simulink model "MOSSE_HDL_final"  (Simulink 8.3)
settings: Solver=FixedStepDiscrete  SolverMode=SingleTasking  StartTime=0.0  StopTime=30*640*360  RelTol=1e-3
InitFcn:
  | %% DSPBuilder Start
  | alt_dspbuilder_update_model(bdroot)
  | %% DSPBuilder End
  | param
StopFcn:
  | % r = rcount.Data(:,:);
  | % w = wcount.Data(:,:);
  | % d = dout.Data(:,:);
  | % ir = read.Data(:,:);
  | % iw = write.Data(:,:);
  | % z = double([ir iw d r w]');
  | %logic_analyzer
values from neighbouring files (symbols this model uses):
  Gau = [4035 -3983 3832 -3589 3269 -2890 2472 -2039 1612 -1211 854 -553 ... (4096 elements, 1x4096)]    [Gauss_coeff.mat]    (also in param.m = reshape(conj(Gau'), 1, 4096))
undefined symbols (not defined in the file or in its folder): gray, psr, source_1, source_2, State_Machine, State_Transition_Table1, window_hann
libraries: allblocks_alteradspbuilder2 x166, hdlsllib x24, hdldemolib x3, simulink x2, dspsigattribs x2, dspmtrx3 x2, visionsinks x1, visiontextngfix x1, dspvision x1
(part 1 of 4)
settings Model: FPTRunName=FPA_Reference  Creator=minimal  LastModifiedBy=minimales
settings DataIOCC: SignalLoggingSaveFormat=Dataset
settings HardwareCC: ProdHWDeviceType=ASIC/FPGA->ASIC/FPGA  TargetIntDivRoundTo=Zero  TargetEndianess=LittleEndian  TargetHWDeviceType=MATLAB Host  ProdEqTarget=off
settings GRTTargetCC: CombineOutputUpdateFcns=on  GRTInterface=off

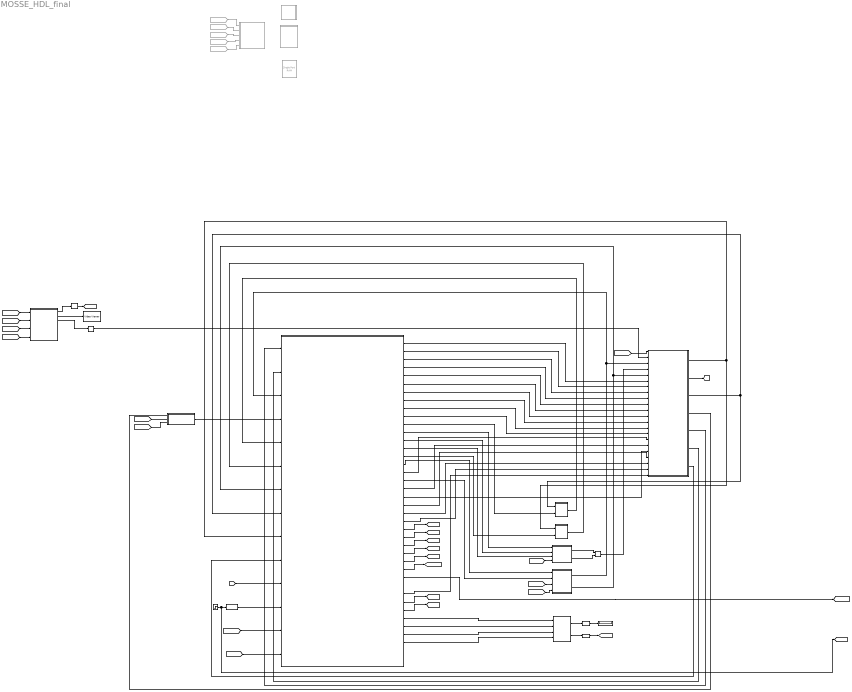
== system MOSSE_HDL_final ==
  DSP_Buider_Alfa_blending_H1 : Subsystem
  DSP_Builder_Alfa_blending_H2 : Subsystem
  DSP_Builder_Compute_PSR : Subsystem  Commented=on
  DSP_Builder_Compute_Shift : Subsystem  Commented=on
  DSP_Builder_Divider Complex : Subsystem
  DSP_Builder_Mult_complex : Subsystem
  DSP_Builder_PSR : Subsystem
  DSP_Builder_Smoothing_Window : Subsystem
  Data Type Conversion1 : DataTypeConversion  OutDataTypeStr=boolean
  Data Type Conversion19 : DataTypeConversion  OutDataTypeStr=int16
  Data Type Conversion5 : DataTypeConversion  OutDataTypeStr=boolean  SampleTime=1
  Delay : Delay  DelayLength=1  InitialCondition=0  SampleTime=1
  Delay1 : Delay  DelayLength=1  InitialCondition=0  SampleTime=1
  Display1 : Display
  From38 : From  Commented=on  GotoTag=source_enb
  From39 : From  Commented=on  GotoTag=source1_enb
  From40 : From  Commented=on  GotoTag=source_control
  From41 : From  Commented=on  GotoTag=source_count_enb
  From42 : From  Commented=on  GotoTag=source_count_rst
  HDL_CODER_Subsystem : Subsystem
  IFFT_res : hdlsllib/HDL Operations/Single Port RAM  Commented=on  ram_size=12  dout_type=New data
  MEM_subsys : Subsystem
  Real-Imag to Complex : RealImagToComplex
  Source : Subsystem  Commented=on
  Step1 : Step  SampleTime=1
  Video Viewer1 : visionsinks/Video Viewer  inputType=Obsolete7b  imagePorts=One multidimensional signal  useColorMap=off  colormapValue=gray(256)  specRange=off  minInputVal=0  maxInputVal=255  FigPos=[1 992 1280 892]  AxisZoom=on  trueSizedOnce=off  OpenAtMdlStart=on  DefaultConfigurationName=vipscopes.VideoViewerScopeCfg
  Video_TestBench : Subsystem
  wires:
  DSP_Builder_Divider Complex/2(Im_r) -> Real-Imag to Complex/2
  DSP_Builder_Divider Complex/1(Re_r) -> Real-Imag to Complex/1
  [rst_win] -> DSP_Builder_Smoothing_Window/2(rst)
  [enb_win] -> DSP_Builder_Smoothing_Window/3(enb)
  [div_complex_aclr] -> DSP_Builder_Divider Complex/4(aclr_i)
  [rst_gauss] -> DSP_Builder_Mult_complex/3(rst)
  [enb_gauss] -> DSP_Builder_Mult_complex/4(enb)
  DSP_Builder_PSR/2(psr_check) -> Data Type Conversion1/1
  Data Type Conversion19/1 -> Display1/1
  Step1/1 -> [enable_tracking], Data Type Conversion5/1
  DSP_Builder_Mult_complex/1(H2) -> MEM_subsys/3(wr_din_F_RAM), HDL_CODER_Subsystem/3("H2 ")
  DSP_Builder_Mult_complex/2(H1) -> MEM_subsys/5(wr_din_G_RAM), HDL_CODER_Subsystem/7(H1)
  DSP_Builder_Smoothing_Window/1(opixel) -> HDL_CODER_Subsystem/4(iPixel_image)
  DSP_Buider_Alfa_blending_H1/1(H) -> HDL_CODER_Subsystem/5(H1_alfa)
  DSP_Builder_Alfa_blending_H2/1(H) -> HDL_CODER_Subsystem/6(H2_alfa)
  [Corr] -> HDL_CODER_Subsystem/11(iCorr_data)
  Data Type Conversion5/1 -> HDL_CODER_Subsystem/12(enable_Tracking)
  [psr_check] -> HDL_CODER_Subsystem/13(psr_check)
  HDL_CODER_Subsystem/11(oData1) -> DSP_Buider_Alfa_blending_H1/2(H_n)
  HDL_CODER_Subsystem/12(Real_H1) -> DSP_Builder_Divider Complex/1(Re_a)
  HDL_CODER_Subsystem/13(Real_H2) -> DSP_Builder_Divider Complex/2(Re_b)
  HDL_CODER_Subsystem/14(Imag_H1) -> DSP_Builder_Divider Complex/3(Im_a)
  HDL_CODER_Subsystem/15(oData2) -> DSP_Builder_Alfa_blending_H2/2(H_n)
  HDL_CODER_Subsystem/16(oF*) -> DSP_Builder_Mult_complex/1(F*)
  HDL_CODER_Subsystem/18(oF) -> DSP_Builder_Mult_complex/2(F)
  HDL_CODER_Subsystem/24(addr_memory_128x128) -> [mem_addr]
  HDL_CODER_Subsystem/25(rst_win) -> [rst_win]
  HDL_CODER_Subsystem/26(enb_win) -> [enb_win]
  HDL_CODER_Subsystem/27(rst_gauss) -> [rst_gauss]
  HDL_CODER_Subsystem/28(enb_gauss) -> [enb_gauss]
  HDL_CODER_Subsystem/29(div_complex) -> [div_complex_aclr]
  HDL_CODER_Subsystem/30(comp_shift_finish) -> [comp_shift_finish]
  [enable_tracking] -> Video_TestBench/1(en)
  [comp_shift_finish] -> Video_TestBench/4(comp_shift_finish)
  Video_TestBench/2(video_viewer) -> Video Viewer1/1
  From40/1 -> Source/1(source_control)
  From38/1 -> Source/2(source_enb)
  From42/1 -> Source/3(source_count_rst)
  From41/1 -> Source/4(source_count_enb)
  From39/1 -> Source/5(source1_enb)
  [enable_write] -> HDL_CODER_Subsystem/14(enable_write)
  [dx] -> Video_TestBench/2(dx)
  [dy] -> Video_TestBench/3(dy)
  Video_TestBench/1(enable_write) -> Delay/1
  Video_TestBench/3(serialized_data) -> Delay1/1
  DSP_Builder_PSR/1(psr) -> Data Type Conversion19/1
  MEM_subsys/3(rd_dout_H1_RAM) -> DSP_Buider_Alfa_blending_H1/1(H_p), HDL_CODER_Subsystem/8(H1_p)
  MEM_subsys/1(rd_dout_H2_RAM) -> DSP_Builder_Alfa_blending_H2/1(H_p), HDL_CODER_Subsystem/9(H2_p)
  [mem_addr] -> MEM_subsys/1(rd_addr_Ext_im_RAM)
  Delay1/1 -> MEM_subsys/2(wr_din_Ext_im_RAM)
  Real-Imag to Complex/1 -> MEM_subsys/4(wr_din_H_RAM)
  HDL_CODER_Subsystem/1(oH2) -> MEM_subsys/6(wr_din_H2_RAM)
  HDL_CODER_Subsystem/2(wr_addr_H1_H2) -> MEM_subsys/7(wr_addr_H1_H2_RAM)
  HDL_CODER_Subsystem/3(we_H1_H2) -> MEM_subsys/8(wr_en_H1_H2_RAM)
  HDL_CODER_Subsystem/4(wr_addr_G_F) -> MEM_subsys/9(wr_addr_G_F_RAM)
  HDL_CODER_Subsystem/5(we_G_F) -> MEM_subsys/10(wr_en_G_F_RAM)
  HDL_CODER_Subsystem/6(addr_in_im) -> MEM_subsys/11(wr_addr_Ext_im_RAM)
  HDL_CODER_Subsystem/7(rd_addr_H1_H2) -> MEM_subsys/12(rd_addr_H1_H2_RAM)
  HDL_CODER_Subsystem/8(rd_addr_G_F) -> MEM_subsys/13(rd_addr_G_F_RAM)
  HDL_CODER_Subsystem/9(we_m) -> MEM_subsys/14(wr_en_Ext_im_RAM)
  HDL_CODER_Subsystem/10(oH1) -> MEM_subsys/15(wr_din_H1_RAM)
  HDL_CODER_Subsystem/17(wr_addr_H) -> MEM_subsys/16(wr_addr_H_RAM)
  HDL_CODER_Subsystem/19(we_H) -> MEM_subsys/17(wr_en_H_RAM)
  HDL_CODER_Subsystem/20(rd_addr_H) -> MEM_subsys/18(rd_addr_H_RAM)
  HDL_CODER_Subsystem/21(RAM_data) -> MEM_subsys/19(wr_din_IFFT_res_RAM)
  HDL_CODER_Subsystem/22(wr_addr_RAM_IFFT) -> MEM_subsys/20(wr_addr_IFFT_res_RAM)
  HDL_CODER_Subsystem/23(we_RAM_IFFT) -> MEM_subsys/21(wr_en_IFFT_res_RAM)
  HDL_CODER_Subsystem/32(rd_addr_RAM_IFFT) -> MEM_subsys/22(rd_addr_IFFT_res_RAM)
  MEM_subsys/2(rd_dout_H_RAM) -> [Corr]
  MEM_subsys/4(rd_dout_Ext_im_RAM) -> DSP_Builder_Smoothing_Window/1(ipixel)
  MEM_subsys/5(rd_dout_G_RAM) -> HDL_CODER_Subsystem/1(G)
  MEM_subsys/6(rd_dout_F_RAM) -> HDL_CODER_Subsystem/2(F)
  MEM_subsys/7(rd_dout_IFFT_res_RAM) -> HDL_CODER_Subsystem/10(In12)
  HDL_CODER_Subsystem/33(Dx) -> [dx]
  HDL_CODER_Subsystem/34(Dy) -> [dy]
  HDL_CODER_Subsystem/35(max_val) -> DSP_Builder_PSR/1(max)
  HDL_CODER_Subsystem/36(mean_val) -> DSP_Builder_PSR/2(mean)
  HDL_CODER_Subsystem/37(tmp_val) -> DSP_Builder_PSR/3(tmp)
  Delay/1 -> [enable_write]
  HDL_CODER_Subsystem/38(psr_reset) -> DSP_Builder_PSR/4(psr_reset)
  Data Type Conversion1/1 -> [psr_check]

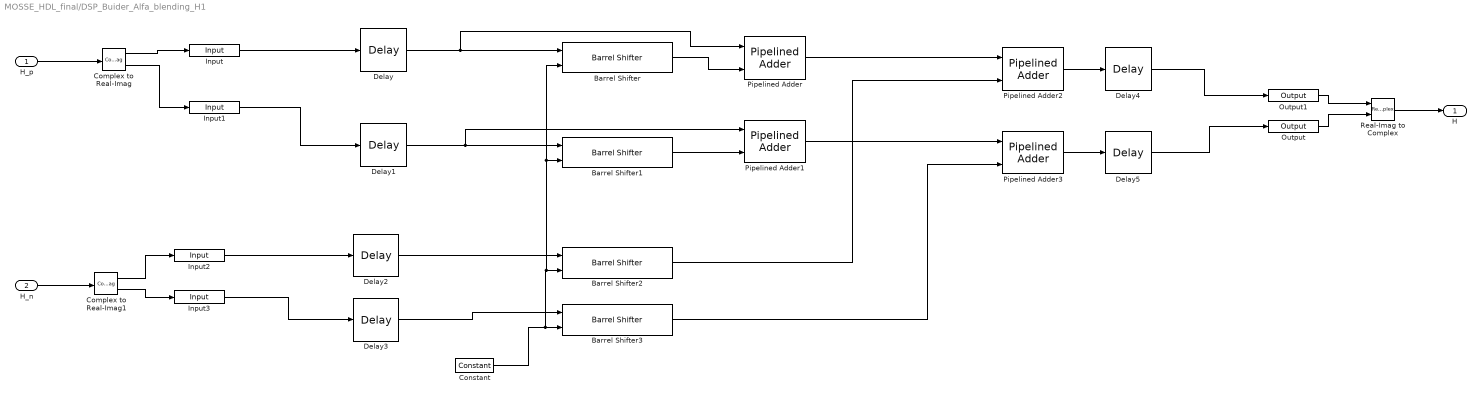
== system MOSSE_HDL_final/DSP_Buider_Alfa_blending_H1 ==
  H_p : Inport
  H_n : Inport  Port=2
  Barrel Shifter : allblocks_alteradspbuilder2/Barrel Shifter  BusType=Signed Integer  bwl=32  bwr=8  pipeline=off  infer_distance=off  distance_length=3  ShiftDirection=Shift right  use_ena=off  use_aclr=off  UseDedicatedCircuitry=off  pipeline_display=0  allowFloatingPointOverride=on  logOutputs=off  logFile=C:\MOSSE%5FHDL%5Ffinal_DSP%5FBuider%5FAlfa%5Fblending%5FH1_Barrel+Shifter.fixedpointlog
  Barrel Shifter1 : allblocks_alteradspbuilder2/Barrel Shifter  BusType=Signed Integer  bwl=32  bwr=8  pipeline=off  infer_distance=off  distance_length=3  ShiftDirection=Shift right  use_ena=off  use_aclr=off  UseDedicatedCircuitry=off  pipeline_display=0  allowFloatingPointOverride=on  logOutputs=off  logFile=E:\Work\ComputerVision\ObjectTrack\MOSSE\autotrackigproject\Model\MOSSE_algorithm\MOSSE_simulink\tb_MOSSE_HDL_final\MOSSE%5FHDL%5Ffinal_DSP%5FBuider%5FAlfa%5Fblending%5FH1_Barrel+Shifter1.fixedpointlog
  Barrel Shifter2 : allblocks_alteradspbuilder2/Barrel Shifter  BusType=Signed Integer  bwl=32  bwr=8  pipeline=off  infer_distance=off  distance_length=3  ShiftDirection=Shift right  use_ena=off  use_aclr=off  UseDedicatedCircuitry=off  pipeline_display=0  allowFloatingPointOverride=on  logOutputs=off  logFile=E:\Work\ComputerVision\ObjectTrack\MOSSE\autotrackigproject\Model\MOSSE_algorithm\MOSSE_simulink\tb_MOSSE_HDL_final\MOSSE%5FHDL%5Ffinal_DSP%5FBuider%5FAlfa%5Fblending%5FH1_Barrel+Shifter2.fixedpointlog
  Barrel Shifter3 : allblocks_alteradspbuilder2/Barrel Shifter  BusType=Signed Integer  bwl=32  bwr=8  pipeline=off  infer_distance=off  distance_length=3  ShiftDirection=Shift right  use_ena=off  use_aclr=off  UseDedicatedCircuitry=off  pipeline_display=0  allowFloatingPointOverride=on  logOutputs=off  logFile=E:\Work\ComputerVision\ObjectTrack\MOSSE\autotrackigproject\Model\MOSSE_algorithm\MOSSE_simulink\tb_MOSSE_HDL_final\MOSSE%5FHDL%5Ffinal_DSP%5FBuider%5FAlfa%5Fblending%5FH1_Barrel+Shifter3.fixedpointlog
  Complex to Real-Imag : ComplexToRealImag
  Complex to Real-Imag1 : ComplexToRealImag
  Constant : allblocks_alteradspbuilder2/Constant  mask_cst=K_shift  BusType=Unsigned Integer  bwl=3  bwr=0  roundMode=Truncate  satMode=Wrap  SpecifyClock=off  allowFloatingPointOverride=on  logOutputs=off  logFile=E:\Work\ComputerVision\ObjectTrack\MOSSE\autotrackigproject\Model\MOSSE_algorithm\MOSSE_simulink\tb_MOSSE_HDL_final\MOSSE%5FHDL%5Ffinal_DSP%5FBuider%5FAlfa%5Fblending%5FH1_Constant.fixedpointlog
  Delay : allblocks_alteradspbuilder2/Delay  pipeline=1  pipeline_display=1  ClockPhase=1  use_ena=off  use_sclr=off  allowFloatingPointOverride=on  logOutputs=off  logFile=E:\Work\ComputerVision\ObjectTrack\MOSSE\autotrackigproject\Model\MOSSE_algorithm\MOSSE_simulink\tb_MOSSE_HDL_final\MOSSE%5FHDL%5Ffinal_DSP%5FBuider%5FAlfa%5Fblending%5FH1_Delay.fixedpointlog  use_init=off  reset_value=1
  Delay1 : allblocks_alteradspbuilder2/Delay  pipeline=1  pipeline_display=1  ClockPhase=1  use_ena=off  use_sclr=off  allowFloatingPointOverride=on  logOutputs=off  logFile=E:\Work\ComputerVision\ObjectTrack\MOSSE\autotrackigproject\Model\MOSSE_algorithm\MOSSE_simulink\tb_MOSSE_HDL_final\MOSSE%5FHDL%5Ffinal_DSP%5FBuider%5FAlfa%5Fblending%5FH1_Delay1.fixedpointlog  use_init=off  reset_value=1
  Delay2 : allblocks_alteradspbuilder2/Delay  pipeline=1  pipeline_display=1  ClockPhase=1  use_ena=off  use_sclr=off  allowFloatingPointOverride=on  logOutputs=off  logFile=E:\Work\ComputerVision\ObjectTrack\MOSSE\autotrackigproject\Model\MOSSE_algorithm\MOSSE_simulink\tb_MOSSE_HDL_final\MOSSE%5FHDL%5Ffinal_DSP%5FBuider%5FAlfa%5Fblending%5FH1_Delay2.fixedpointlog  use_init=off  reset_value=1
  Delay3 : allblocks_alteradspbuilder2/Delay  pipeline=1  pipeline_display=1  ClockPhase=1  use_ena=off  use_sclr=off  allowFloatingPointOverride=on  logOutputs=off  logFile=E:\Work\ComputerVision\ObjectTrack\MOSSE\autotrackigproject\Model\MOSSE_algorithm\MOSSE_simulink\tb_MOSSE_HDL_final\MOSSE%5FHDL%5Ffinal_DSP%5FBuider%5FAlfa%5Fblending%5FH1_Delay3.fixedpointlog  use_init=off  reset_value=1
  Delay4 : allblocks_alteradspbuilder2/Delay  pipeline=1  pipeline_display=1  ClockPhase=1  use_ena=off  use_sclr=off  allowFloatingPointOverride=on  logOutputs=off  logFile=E:\Work\ComputerVision\ObjectTrack\MOSSE\autotrackigproject\Model\MOSSE_algorithm\MOSSE_simulink\tb_MOSSE_HDL_final\MOSSE%5FHDL%5Ffinal_DSP%5FBuider%5FAlfa%5Fblending%5FH1_Delay4.fixedpointlog  use_init=off  reset_value=1
  Delay5 : allblocks_alteradspbuilder2/Delay  pipeline=1  pipeline_display=1  ClockPhase=1  use_ena=off  use_sclr=off  allowFloatingPointOverride=on  logOutputs=off  logFile=E:\Work\ComputerVision\ObjectTrack\MOSSE\autotrackigproject\Model\MOSSE_algorithm\MOSSE_simulink\tb_MOSSE_HDL_final\MOSSE%5FHDL%5Ffinal_DSP%5FBuider%5FAlfa%5Fblending%5FH1_Delay5.fixedpointlog  use_init=off  reset_value=1
  Input : allblocks_alteradspbuilder2/Input  iofile=E:\Work\ComputerVision\ObjectTrack\MOSSE\autotrackigproject\Model\MOSSE_algorithm\MOSSE_simulink\tb_MOSSE_HDL_final\MOSSE%5FHDL%5Ffinal_DSP%5FBuider%5FAlfa%5Fblending%5FH1_Input.salt  BusType=Signed Integer  bwl=32  bwr=0  SpecifyClock=off  PORTTYPE=Input  externalType=Inferred  allowFloatingPointOverride=on  logOutputs=off
  Input1 : allblocks_alteradspbuilder2/Input  iofile=E:\Work\ComputerVision\ObjectTrack\MOSSE\autotrackigproject\Model\MOSSE_algorithm\MOSSE_simulink\tb_MOSSE_HDL_final\MOSSE%5FHDL%5Ffinal_DSP%5FBuider%5FAlfa%5Fblending%5FH1_Input1.salt  BusType=Signed Integer  bwl=32  bwr=0  SpecifyClock=off  PORTTYPE=Input  externalType=Inferred  allowFloatingPointOverride=on  logOutputs=off
  Input2 : allblocks_alteradspbuilder2/Input  iofile=E:\Work\ComputerVision\ObjectTrack\MOSSE\autotrackigproject\Model\MOSSE_algorithm\MOSSE_simulink\tb_MOSSE_HDL_final\MOSSE%5FHDL%5Ffinal_DSP%5FBuider%5FAlfa%5Fblending%5FH1_Input2.salt  BusType=Signed Integer  bwl=32  bwr=0  SpecifyClock=off  PORTTYPE=Input  externalType=Inferred  allowFloatingPointOverride=on  logOutputs=off
  Input3 : allblocks_alteradspbuilder2/Input  iofile=E:\Work\ComputerVision\ObjectTrack\MOSSE\autotrackigproject\Model\MOSSE_algorithm\MOSSE_simulink\tb_MOSSE_HDL_final\MOSSE%5FHDL%5Ffinal_DSP%5FBuider%5FAlfa%5Fblending%5FH1_Input3.salt  BusType=Signed Integer  bwl=32  bwr=0  SpecifyClock=off  PORTTYPE=Input  externalType=Inferred  allowFloatingPointOverride=on  logOutputs=off
  Output : allblocks_alteradspbuilder2/Output  iofile=E:\Work\ComputerVision\ObjectTrack\MOSSE\autotrackigproject\Model\MOSSE_algorithm\MOSSE_simulink\tb_MOSSE_HDL_final\MOSSE%5FHDL%5Ffinal_DSP%5FBuider%5FAlfa%5Fblending%5FH1_Output.capture  BusType=Signed Integer  bwl=32  bwr=0  externalType=Simulink Fixed Point Type  PORTTYPE=Output  allowFloatingPointOverride=on  logOutputs=off
  Output1 : allblocks_alteradspbuilder2/Output  iofile=E:\Work\ComputerVision\ObjectTrack\MOSSE\autotrackigproject\Model\MOSSE_algorithm\MOSSE_simulink\tb_MOSSE_HDL_final\MOSSE%5FHDL%5Ffinal_DSP%5FBuider%5FAlfa%5Fblending%5FH1_Output1.capture  BusType=Signed Integer  bwl=32  bwr=0  externalType=Simulink Fixed Point Type  PORTTYPE=Output  allowFloatingPointOverride=on  logOutputs=off
  Pipelined Adder : allblocks_alteradspbuilder2/Pipelined Adder  BusType=Signed Integer  bwl=32  bwr=0  pipeline=0  pipeline_display=0  AddSubDirection=SUB  use_cin=off  use_ovl=off  use_addsub=off  use_ena=off  use_aclr=off  or_aclr_inputs=on
  Pipelined Adder1 : allblocks_alteradspbuilder2/Pipelined Adder  BusType=Signed Integer  bwl=32  bwr=0  pipeline=0  pipeline_display=0  AddSubDirection=SUB  use_cin=off  use_ovl=off  use_addsub=off  use_ena=off  use_aclr=off  or_aclr_inputs=on
  Pipelined Adder2 : allblocks_alteradspbuilder2/Pipelined Adder  BusType=Signed Integer  bwl=32  bwr=0  pipeline=0  pipeline_display=0  AddSubDirection=ADD  use_cin=off  use_ovl=off  use_addsub=off  use_ena=off  use_aclr=off  or_aclr_inputs=on
  Pipelined Adder3 : allblocks_alteradspbuilder2/Pipelined Adder  BusType=Signed Integer  bwl=32  bwr=0  pipeline=0  pipeline_display=0  AddSubDirection=ADD  use_cin=off  use_ovl=off  use_addsub=off  use_ena=off  use_aclr=off  or_aclr_inputs=on
  Real-Imag to Complex : RealImagToComplex
  H : Outport
  wires:
  Pipelined Adder/1 -> Pipelined Adder2/1
  Barrel Shifter/1 -> Pipelined Adder/2
  Barrel Shifter2/1 -> Pipelined Adder2/2
  Barrel Shifter3/1 -> Pipelined Adder3/2
  Pipelined Adder1/1 -> Pipelined Adder3/1
  Barrel Shifter1/1 -> Pipelined Adder1/2
  H_p/1 -> Complex to Real-Imag/1
  H_n/1 -> Complex to Real-Imag1/1
  Real-Imag to Complex/1 -> H/1
  Constant/1 -> Barrel Shifter/2, Barrel Shifter1/2, Barrel Shifter2/2, Barrel Shifter3/2
  Complex to Real-Imag/1 -> Input/1
  Complex to Real-Imag/2 -> Input1/1
  Complex to Real-Imag1/1 -> Input2/1
  Complex to Real-Imag1/2 -> Input3/1
  Input/1 -> Delay/1
  Delay/1 -> Pipelined Adder/1, Barrel Shifter/1
  Input1/1 -> Delay1/1
  Delay1/1 -> Pipelined Adder1/1, Barrel Shifter1/1
  Input2/1 -> Delay2/1
  Delay2/1 -> Barrel Shifter2/1
  Input3/1 -> Delay3/1
  Delay3/1 -> Barrel Shifter3/1
  Output1/1 -> Real-Imag to Complex/1
  Output/1 -> Real-Imag to Complex/2
  Pipelined Adder2/1 -> Delay4/1
  Delay4/1 -> Output1/1
  Pipelined Adder3/1 -> Delay5/1
  Delay5/1 -> Output/1

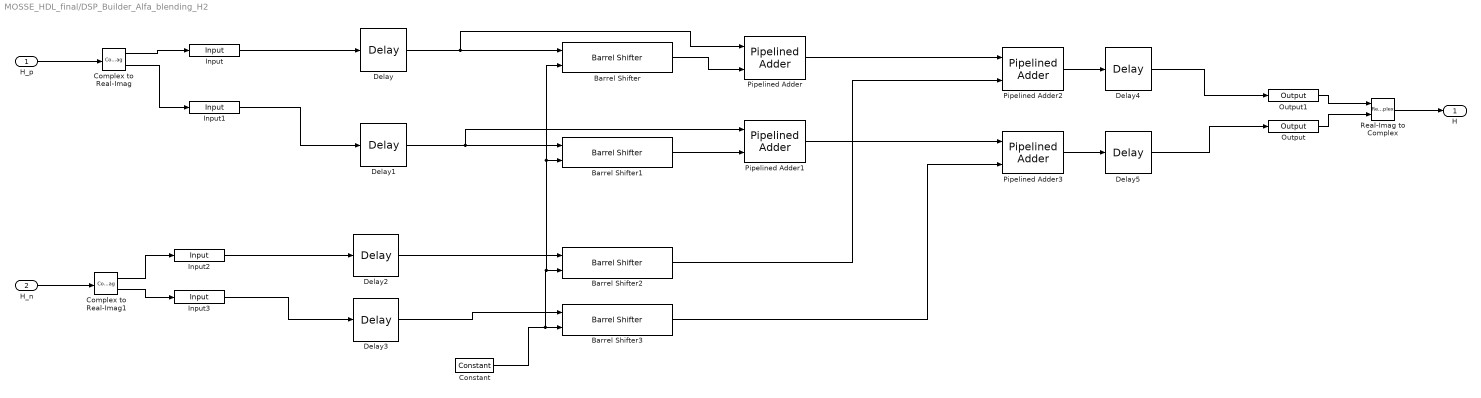
== system MOSSE_HDL_final/DSP_Builder_Alfa_blending_H2 ==
  H_p : Inport
  H_n : Inport  Port=2
  Barrel Shifter : allblocks_alteradspbuilder2/Barrel Shifter  BusType=Signed Integer  bwl=32  bwr=8  pipeline=off  infer_distance=off  distance_length=3  ShiftDirection=Shift right  use_ena=off  use_aclr=off  UseDedicatedCircuitry=off  pipeline_display=0  allowFloatingPointOverride=on  logOutputs=off  logFile=E:\Work\ComputerVision\ObjectTrack\MOSSE\autotrackigproject\Model\MOSSE_algorithm\MOSSE_simulink\tb_MOSSE_HDL_final\MOSSE%5FHDL%5Ffinal_DSP%5FBuilder%5FAlfa%5Fblending%5FH2_Barrel+Shifter.fixedpointlog
  Barrel Shifter1 : allblocks_alteradspbuilder2/Barrel Shifter  BusType=Signed Integer  bwl=32  bwr=8  pipeline=off  infer_distance=off  distance_length=3  ShiftDirection=Shift right  use_ena=off  use_aclr=off  UseDedicatedCircuitry=off  pipeline_display=0  allowFloatingPointOverride=on  logOutputs=off  logFile=E:\Work\ComputerVision\ObjectTrack\MOSSE\autotrackigproject\Model\MOSSE_algorithm\MOSSE_simulink\tb_MOSSE_HDL_final\MOSSE%5FHDL%5Ffinal_DSP%5FBuilder%5FAlfa%5Fblending%5FH2_Barrel+Shifter1.fixedpointlog
  Barrel Shifter2 : allblocks_alteradspbuilder2/Barrel Shifter  BusType=Signed Integer  bwl=32  bwr=8  pipeline=off  infer_distance=off  distance_length=3  ShiftDirection=Shift right  use_ena=off  use_aclr=off  UseDedicatedCircuitry=off  pipeline_display=0  allowFloatingPointOverride=on  logOutputs=off  logFile=E:\Work\ComputerVision\ObjectTrack\MOSSE\autotrackigproject\Model\MOSSE_algorithm\MOSSE_simulink\tb_MOSSE_HDL_final\MOSSE%5FHDL%5Ffinal_DSP%5FBuilder%5FAlfa%5Fblending%5FH2_Barrel+Shifter2.fixedpointlog
  Barrel Shifter3 : allblocks_alteradspbuilder2/Barrel Shifter  BusType=Signed Integer  bwl=32  bwr=8  pipeline=off  infer_distance=off  distance_length=3  ShiftDirection=Shift right  use_ena=off  use_aclr=off  UseDedicatedCircuitry=off  pipeline_display=0  allowFloatingPointOverride=on  logOutputs=off  logFile=E:\Work\ComputerVision\ObjectTrack\MOSSE\autotrackigproject\Model\MOSSE_algorithm\MOSSE_simulink\tb_MOSSE_HDL_final\MOSSE%5FHDL%5Ffinal_DSP%5FBuilder%5FAlfa%5Fblending%5FH2_Barrel+Shifter3.fixedpointlog
  Complex to Real-Imag : ComplexToRealImag
  Complex to Real-Imag1 : ComplexToRealImag
  Constant : allblocks_alteradspbuilder2/Constant  mask_cst=K_shift  BusType=Unsigned Integer  bwl=3  bwr=0  roundMode=Truncate  satMode=Wrap  SpecifyClock=off  allowFloatingPointOverride=on  logOutputs=off  logFile=E:\Work\ComputerVision\ObjectTrack\MOSSE\autotrackigproject\Model\MOSSE_algorithm\MOSSE_simulink\tb_MOSSE_HDL_final\MOSSE%5FHDL%5Ffinal_DSP%5FBuilder%5FAlfa%5Fblending%5FH2_Constant.fixedpointlog
  Delay : allblocks_alteradspbuilder2/Delay  pipeline=1  pipeline_display=1  ClockPhase=1  use_ena=off  use_sclr=off  allowFloatingPointOverride=on  logOutputs=off  logFile=E:\Work\ComputerVision\ObjectTrack\MOSSE\autotrackigproject\Model\MOSSE_algorithm\MOSSE_simulink\tb_MOSSE_HDL_final\MOSSE%5FHDL%5Ffinal_DSP%5FBuilder%5FAlfa%5Fblending%5FH2_Delay.fixedpointlog  use_init=off  reset_value=1
  Delay1 : allblocks_alteradspbuilder2/Delay  pipeline=1  pipeline_display=1  ClockPhase=1  use_ena=off  use_sclr=off  allowFloatingPointOverride=on  logOutputs=off  logFile=E:\Work\ComputerVision\ObjectTrack\MOSSE\autotrackigproject\Model\MOSSE_algorithm\MOSSE_simulink\tb_MOSSE_HDL_final\MOSSE%5FHDL%5Ffinal_DSP%5FBuilder%5FAlfa%5Fblending%5FH2_Delay1.fixedpointlog  use_init=off  reset_value=1
  Delay2 : allblocks_alteradspbuilder2/Delay  pipeline=1  pipeline_display=1  ClockPhase=1  use_ena=off  use_sclr=off  allowFloatingPointOverride=on  logOutputs=off  logFile=E:\Work\ComputerVision\ObjectTrack\MOSSE\autotrackigproject\Model\MOSSE_algorithm\MOSSE_simulink\tb_MOSSE_HDL_final\MOSSE%5FHDL%5Ffinal_DSP%5FBuilder%5FAlfa%5Fblending%5FH2_Delay2.fixedpointlog  use_init=off  reset_value=1
  Delay3 : allblocks_alteradspbuilder2/Delay  pipeline=1  pipeline_display=1  ClockPhase=1  use_ena=off  use_sclr=off  allowFloatingPointOverride=on  logOutputs=off  logFile=E:\Work\ComputerVision\ObjectTrack\MOSSE\autotrackigproject\Model\MOSSE_algorithm\MOSSE_simulink\tb_MOSSE_HDL_final\MOSSE%5FHDL%5Ffinal_DSP%5FBuilder%5FAlfa%5Fblending%5FH2_Delay3.fixedpointlog  use_init=off  reset_value=1
  Delay4 : allblocks_alteradspbuilder2/Delay  pipeline=1  pipeline_display=1  ClockPhase=1  use_ena=off  use_sclr=off  allowFloatingPointOverride=on  logOutputs=off  logFile=E:\Work\ComputerVision\ObjectTrack\MOSSE\autotrackigproject\Model\MOSSE_algorithm\MOSSE_simulink\tb_MOSSE_HDL_final\MOSSE%5FHDL%5Ffinal_DSP%5FBuilder%5FAlfa%5Fblending%5FH2_Delay4.fixedpointlog  use_init=off  reset_value=1
  Delay5 : allblocks_alteradspbuilder2/Delay  pipeline=1  pipeline_display=1  ClockPhase=1  use_ena=off  use_sclr=off  allowFloatingPointOverride=on  logOutputs=off  logFile=E:\Work\ComputerVision\ObjectTrack\MOSSE\autotrackigproject\Model\MOSSE_algorithm\MOSSE_simulink\tb_MOSSE_HDL_final\MOSSE%5FHDL%5Ffinal_DSP%5FBuilder%5FAlfa%5Fblending%5FH2_Delay5.fixedpointlog  use_init=off  reset_value=1
  Input : allblocks_alteradspbuilder2/Input  iofile=E:\Work\ComputerVision\ObjectTrack\MOSSE\autotrackigproject\Model\MOSSE_algorithm\MOSSE_simulink\tb_MOSSE_HDL_final\MOSSE%5FHDL%5Ffinal_DSP%5FBuilder%5FAlfa%5Fblending%5FH2_Input.salt  BusType=Signed Integer  bwl=32  bwr=0  SpecifyClock=off  PORTTYPE=Input  externalType=Inferred  allowFloatingPointOverride=on  logOutputs=off
  Input1 : allblocks_alteradspbuilder2/Input  iofile=E:\Work\ComputerVision\ObjectTrack\MOSSE\autotrackigproject\Model\MOSSE_algorithm\MOSSE_simulink\tb_MOSSE_HDL_final\MOSSE%5FHDL%5Ffinal_DSP%5FBuilder%5FAlfa%5Fblending%5FH2_Input1.salt  BusType=Signed Integer  bwl=32  bwr=0  SpecifyClock=off  PORTTYPE=Input  externalType=Inferred  allowFloatingPointOverride=on  logOutputs=off
  Input2 : allblocks_alteradspbuilder2/Input  iofile=E:\Work\ComputerVision\ObjectTrack\MOSSE\autotrackigproject\Model\MOSSE_algorithm\MOSSE_simulink\tb_MOSSE_HDL_final\MOSSE%5FHDL%5Ffinal_DSP%5FBuilder%5FAlfa%5Fblending%5FH2_Input2.salt  BusType=Signed Integer  bwl=32  bwr=0  SpecifyClock=off  PORTTYPE=Input  externalType=Inferred  allowFloatingPointOverride=on  logOutputs=off
  Input3 : allblocks_alteradspbuilder2/Input  iofile=E:\Work\ComputerVision\ObjectTrack\MOSSE\autotrackigproject\Model\MOSSE_algorithm\MOSSE_simulink\tb_MOSSE_HDL_final\MOSSE%5FHDL%5Ffinal_DSP%5FBuilder%5FAlfa%5Fblending%5FH2_Input3.salt  BusType=Signed Integer  bwl=32  bwr=0  SpecifyClock=off  PORTTYPE=Input  externalType=Inferred  allowFloatingPointOverride=on  logOutputs=off
  Output : allblocks_alteradspbuilder2/Output  iofile=E:\Work\ComputerVision\ObjectTrack\MOSSE\autotrackigproject\Model\MOSSE_algorithm\MOSSE_simulink\tb_MOSSE_HDL_final\MOSSE%5FHDL%5Ffinal_DSP%5FBuilder%5FAlfa%5Fblending%5FH2_Output.capture  BusType=Signed Integer  bwl=32  bwr=0  externalType=Simulink Fixed Point Type  PORTTYPE=Output  allowFloatingPointOverride=on  logOutputs=off
  Output1 : allblocks_alteradspbuilder2/Output  iofile=E:\Work\ComputerVision\ObjectTrack\MOSSE\autotrackigproject\Model\MOSSE_algorithm\MOSSE_simulink\tb_MOSSE_HDL_final\MOSSE%5FHDL%5Ffinal_DSP%5FBuilder%5FAlfa%5Fblending%5FH2_Output1.capture  BusType=Signed Integer  bwl=32  bwr=0  externalType=Simulink Fixed Point Type  PORTTYPE=Output  allowFloatingPointOverride=on  logOutputs=off
  Pipelined Adder : allblocks_alteradspbuilder2/Pipelined Adder  BusType=Signed Integer  bwl=32  bwr=0  pipeline=0  pipeline_display=0  AddSubDirection=SUB  use_cin=off  use_ovl=off  use_addsub=off  use_ena=off  use_aclr=off  or_aclr_inputs=on
  Pipelined Adder1 : allblocks_alteradspbuilder2/Pipelined Adder  BusType=Signed Integer  bwl=32  bwr=0  pipeline=0  pipeline_display=0  AddSubDirection=SUB  use_cin=off  use_ovl=off  use_addsub=off  use_ena=off  use_aclr=off  or_aclr_inputs=on
  Pipelined Adder2 : allblocks_alteradspbuilder2/Pipelined Adder  BusType=Signed Integer  bwl=32  bwr=0  pipeline=0  pipeline_display=0  AddSubDirection=ADD  use_cin=off  use_ovl=off  use_addsub=off  use_ena=off  use_aclr=off  or_aclr_inputs=on
  Pipelined Adder3 : allblocks_alteradspbuilder2/Pipelined Adder  BusType=Signed Integer  bwl=32  bwr=0  pipeline=0  pipeline_display=0  AddSubDirection=ADD  use_cin=off  use_ovl=off  use_addsub=off  use_ena=off  use_aclr=off  or_aclr_inputs=on
  Real-Imag to Complex : RealImagToComplex
  H : Outport
  wires:
  Pipelined Adder/1 -> Pipelined Adder2/1
  Barrel Shifter/1 -> Pipelined Adder/2
  Barrel Shifter2/1 -> Pipelined Adder2/2
  Barrel Shifter3/1 -> Pipelined Adder3/2
  Pipelined Adder1/1 -> Pipelined Adder3/1
  Barrel Shifter1/1 -> Pipelined Adder1/2
  H_p/1 -> Complex to Real-Imag/1
  H_n/1 -> Complex to Real-Imag1/1
  Real-Imag to Complex/1 -> H/1
  Constant/1 -> Barrel Shifter/2, Barrel Shifter1/2, Barrel Shifter2/2, Barrel Shifter3/2
  Complex to Real-Imag/1 -> Input/1
  Complex to Real-Imag/2 -> Input1/1
  Complex to Real-Imag1/1 -> Input2/1
  Complex to Real-Imag1/2 -> Input3/1
  Input/1 -> Delay/1
  Delay/1 -> Pipelined Adder/1, Barrel Shifter/1
  Input1/1 -> Delay1/1
  Delay1/1 -> Pipelined Adder1/1, Barrel Shifter1/1
  Input2/1 -> Delay2/1
  Delay2/1 -> Barrel Shifter2/1
  Input3/1 -> Delay3/1
  Delay3/1 -> Barrel Shifter3/1
  Output1/1 -> Real-Imag to Complex/1
  Output/1 -> Real-Imag to Complex/2
  Pipelined Adder2/1 -> Delay4/1
  Delay4/1 -> Output1/1
  Pipelined Adder3/1 -> Delay5/1
  Delay5/1 -> Output/1

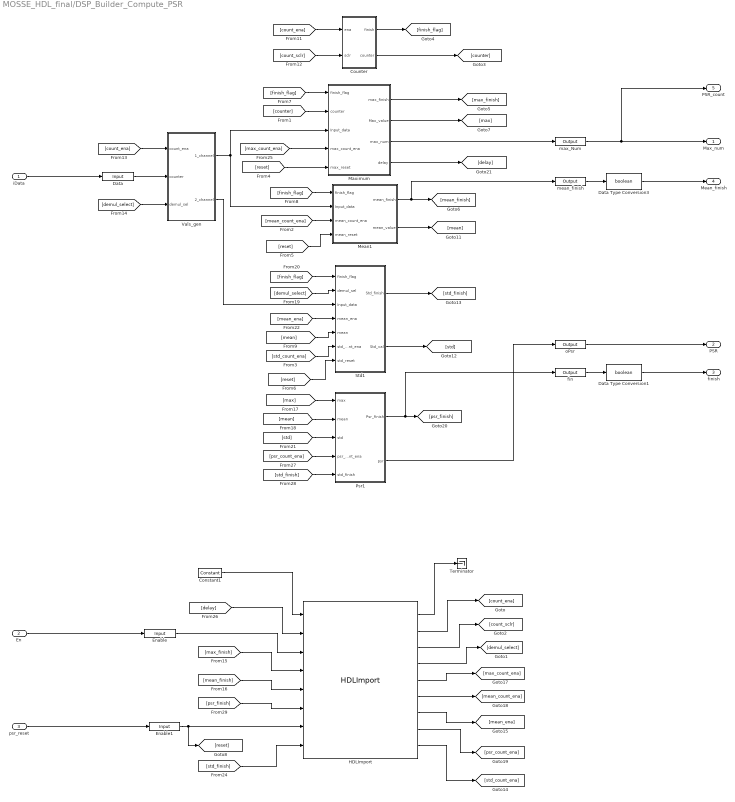
== system MOSSE_HDL_final/DSP_Builder_Compute_PSR ==
  iData : Inport
  En : Inport  Port=2
  psr_reset : Inport  Port=3
  Constant1 : allblocks_alteradspbuilder2/Constant  mask_cst=1  BusType=Single Bit  bwl=8  bwr=0  roundMode=Truncate  satMode=Wrap  SpecifyClock=off  allowFloatingPointOverride=on  logOutputs=off  logFile=d:\Project\AutoTracking\model\MOSSE_work\MOSSE_model\MOSSE_Final_models\tb_MOSSE_HDL_final\MOSSE%5FHDL%5Ffinal_DSP%5FBuilder%5FCompute%5FPSR_Constant1.fixedpointlog
  Counter : Subsystem
  Data : allblocks_alteradspbuilder2/Input  iofile=d:\Project\AutoTracking\model\MOSSE_work\MOSSE_model\MOSSE_Final_models\tb_MOSSE_HDL_final\MOSSE%5FHDL%5Ffinal_DSP%5FBuilder%5FCompute%5FPSR_Data.salt  BusType=Signed Integer  bwl=16  bwr=0  SpecifyClock=off  PORTTYPE=Input  externalType=Inferred  allowFloatingPointOverride=on  logOutputs=off
  Data Type Conversion1 : DataTypeConversion  OutDataTypeStr=boolean
  Data Type Conversion3 : DataTypeConversion  OutDataTypeStr=boolean
  Enable : allblocks_alteradspbuilder2/Input  iofile=d:\Project\AutoTracking\model\MOSSE_work\MOSSE_model\MOSSE_Final_models\tb_MOSSE_HDL_final\MOSSE%5FHDL%5Ffinal_DSP%5FBuilder%5FCompute%5FPSR_Enable.salt  BusType=Single Bit  bwl=16  bwr=0  SpecifyClock=off  PORTTYPE=Input  externalType=Inferred  allowFloatingPointOverride=on  logOutputs=off
  Enable1 : allblocks_alteradspbuilder2/Input  iofile=d:\Project\AutoTracking\model\MOSSE_work\MOSSE_model\MOSSE_Final_models\tb_MOSSE_HDL_final\MOSSE%5FHDL%5Ffinal_DSP%5FBuilder%5FCompute%5FPSR_Enable1.salt  BusType=Single Bit  bwl=16  bwr=0  SpecifyClock=off  PORTTYPE=Input  externalType=Inferred  allowFloatingPointOverride=on  logOutputs=off
  HDLImport : allblocks_alteradspbuilder2/HDLImport  entityName=State_Machine_import  inNames=clk_enable delay enable_in max_finish mean_finish psr_finish reset std_finish  inBwls=1 1 1 1 1 1 1 1  inBwrs="0  0  0  0  0  0  0  0"  inTypes=b b b b b b b b  inDelayed="0  0  0  0  0  0  0  0"  outNames=ce_out count_ena count_sclr demul_select max_count_ena mean_count_ena mean_ena psr_count_ena std_count_ena  outBwls=1 1 1 1 1 1 1 1 1  outBwrs="0  0  0  0  0  0  0  0  0"  outTypes=b b b b b b b b b  xmlmapfile=C:\altera\13.0\quartus\dsp_builder\lib\SimgenCMap.xml  vofile=DSPBuilder_MOSSE_HDL_final_import\State_Machine.vo  src_file=psr\State_Machine.v;psr\State_Transition_Table1.v;  TopLevelName=State_Machine  UseQPF=0  n_input_port=8  n_output_port=9  array_clocks=clk  use_systemC_model=off  is_megacore=off  use_dynamic_feedthrough_data=off  use_alphabetical_port_ordering=on  allowFloatingPointOverride=off
  Maximum : Subsystem
  Mean1 : Subsystem
  Psr1 : Subsystem
  Std1 : Subsystem
  Terminator : Terminator
  Vals_gen : Subsystem
  fin : allblocks_alteradspbuilder2/Output  iofile=d:\Project\AutoTracking\model\MOSSE_work\MOSSE_model\MOSSE_Final_models\tb_MOSSE_HDL_final\MOSSE%5FHDL%5Ffinal_DSP%5FBuilder%5FCompute%5FPSR_fin.capture  BusType=Single Bit  bwl=32  bwr=0  externalType=Simulink Fixed Point Type  PORTTYPE=Output  allowFloatingPointOverride=on  logOutputs=off
  max_Num : allblocks_alteradspbuilder2/Output  iofile=d:\Project\AutoTracking\model\MOSSE_work\MOSSE_model\MOSSE_Final_models\tb_MOSSE_HDL_final\MOSSE%5FHDL%5Ffinal_DSP%5FBuilder%5FCompute%5FPSR_max%5FNum.capture  BusType=Signed Integer  bwl=16  bwr=0  externalType=Simulink Fixed Point Type  PORTTYPE=Output  allowFloatingPointOverride=on  logOutputs=off
  mean_finish : allblocks_alteradspbuilder2/Output  iofile=d:\Project\AutoTracking\model\MOSSE_work\MOSSE_model\MOSSE_Final_models\tb_MOSSE_HDL_final\MOSSE%5FHDL%5Ffinal_DSP%5FBuilder%5FCompute%5FPSR_mean%5Ffinish.capture  BusType=Single Bit  bwl=16  bwr=0  externalType=Simulink Fixed Point Type  PORTTYPE=Output  allowFloatingPointOverride=on  logOutputs=off
  oPsr : allblocks_alteradspbuilder2/Output  iofile=d:\Project\AutoTracking\model\MOSSE_work\MOSSE_model\MOSSE_Final_models\tb_MOSSE_HDL_final\MOSSE%5FHDL%5Ffinal_DSP%5FBuilder%5FCompute%5FPSR_oPsr.capture  BusType=Signed Integer  bwl=32  bwr=0  externalType=Simulink Fixed Point Type  PORTTYPE=Output  allowFloatingPointOverride=on  logOutputs=off
  Max_num : Outport
  PSR : Outport  Port=2
  finish : Outport  Port=3
  Mean_finish : Outport  Port=4
  PSR_count : Outport  Port=5
  wires:
  [demul_select] -> Std1/2(demul_sel)
  Data/1 -> Vals_gen/2(counter)
  [demul_select] -> Vals_gen/3(demul_sel)
  Vals_gen/2(2_channel) -> Std1/3(Input_data)
  [finish_flag] -> Std1/1(finish_flag)
  Std1/1(Std_finish) -> [std_finish]
  Mean1/2(mean_value) -> [mean]
  max_Num/1 -> PSR_count/1, Max_num/1
  Maximum/2(Max_value) -> [max]
  [mean] -> Std1/5(mean)
  [mean_ena] -> Std1/4(mean_ena)
  [max] -> Psr1/1(max)
  Maximum/4(delay) -> [delay]
  HDLImport/1 -> Terminator/1
  Constant1/1 -> HDLImport/1
  [psr_finish] -> HDLImport/6
  [std_finish] -> HDLImport/8
  [mean_finish] -> HDLImport/5
  [max_finish] -> HDLImport/4
  [delay] -> HDLImport/2
  Mean1/1(mean_finish) -> mean_finish/1, [mean_finish]
  oPsr/1 -> PSR/1
  [count_ena] -> Vals_gen/1(count_ena)
  Psr1/1(Psr_finish) -> fin/1, [psr_finish]
  Vals_gen/1(1_channel) -> Maximum/3(Input_data), Mean1/2(Input_data)
  [mean_count_ena] -> Mean1/3(mean_count_ena)
  Counter/1(finish) -> [finish_flag]
  Maximum/1(max_finish) -> [max_finish]
  [counter] -> Maximum/2(counter)
  [finish_flag] -> Maximum/1(finish_flag)
  [finish_flag] -> Mean1/1(finish_flag)
  [count_ena] -> Counter/1(ena)
  [count_sclr] -> Counter/2(sclr)
  [std_finish] -> Psr1/5(std_finish)
  Psr1/2(psr) -> oPsr/1
  [mean] -> Psr1/2(mean)
  [std] -> Psr1/3(std)
  Std1/2(Std_val) -> [std]
  [std_count_ena] -> Std1/6(std_count_ena)
  [psr_count_ena] -> Psr1/4(psr_count_ena)
  [max_count_ena] -> Maximum/4(max_count_ena)
  HDLImport/3 -> [count_sclr]
  HDLImport/2 -> [count_ena]
  HDLImport/6 -> [mean_count_ena]
  Enable/1 -> HDLImport/3
  HDLImport/4 -> [demul_select]
  HDLImport/5 -> [max_count_ena]
  HDLImport/7 -> [mean_ena]
  HDLImport/8 -> [psr_count_ena]
  HDLImport/9 -> [std_count_ena]
  Counter/2(counter) -> [counter]
  En/1 -> Enable/1
  iData/1 -> Data/1
  psr_reset/1 -> Enable1/1
  Enable1/1 -> [reset], HDLImport/7
  mean_finish/1 -> Data Type Conversion3/1
  fin/1 -> Data Type Conversion1/1
  Data Type Conversion1/1 -> finish/1
  Data Type Conversion3/1 -> Mean_finish/1
  [reset] -> Maximum/5(max_reset)
  [reset] -> Mean1/4(mean_reset)
  [reset] -> Std1/7(std_reset)
  Maximum/3(max_num) -> max_Num/1

== system MOSSE_HDL_final/DSP_Builder_Compute_Shift ==
  In_num : Inport
  iaclr : Inport  Port=2
  Constant : allblocks_alteradspbuilder2/Constant  mask_cst=64  BusType=Unsigned Integer  bwl=8  bwr=0  roundMode=Truncate  satMode=Wrap  SpecifyClock=off  allowFloatingPointOverride=on  logOutputs=off  logFile=C:\Workspace\Autotracking\MOSSE_model\tb_MOSSE_HDL_final\MOSSE%5FHDL%5Ffinal_DSP%5FBuilder%5FCompute%5FShift_Constant.fixedpointlog
  Constant1 : allblocks_alteradspbuilder2/Constant  mask_cst=31  BusType=Signed Integer  bwl=8  bwr=0  roundMode=Truncate  satMode=Wrap  SpecifyClock=off  allowFloatingPointOverride=on  logOutputs=off  logFile=C:\Workspace\Autotracking\MOSSE_model\tb_MOSSE_HDL_final\MOSSE%5FHDL%5Ffinal_DSP%5FBuilder%5FCompute%5FShift_Constant1.fixedpointlog
  Constant2 : allblocks_alteradspbuilder2/Constant  mask_cst=32  BusType=Signed Integer  bwl=8  bwr=0  roundMode=Truncate  satMode=Wrap  SpecifyClock=off  allowFloatingPointOverride=on  logOutputs=off  logFile=C:\Workspace\Autotracking\MOSSE_model\tb_MOSSE_HDL_final\MOSSE%5FHDL%5Ffinal_DSP%5FBuilder%5FCompute%5FShift_Constant2.fixedpointlog
  Delay : allblocks_alteradspbuilder2/Delay  pipeline=1  pipeline_display=1  ClockPhase=1  use_ena=off  use_sclr=on  allowFloatingPointOverride=on  logOutputs=off  logFile=C:\Workspace\Autotracking\MOSSE_model\tb_MOSSE_HDL_final\MOSSE%5FHDL%5Ffinal_DSP%5FBuilder%5FCompute%5FShift_Delay.fixedpointlog  use_init=off  reset_value=1
  Delay1 : allblocks_alteradspbuilder2/Delay  pipeline=1  pipeline_display=1  ClockPhase=1  use_ena=off  use_sclr=on  allowFloatingPointOverride=on  logOutputs=off  logFile=C:\Workspace\Autotracking\MOSSE_model\tb_MOSSE_HDL_final\MOSSE%5FHDL%5Ffinal_DSP%5FBuilder%5FCompute%5FShift_Delay1.fixedpointlog  use_init=off  reset_value=1
  Delay2 : allblocks_alteradspbuilder2/Delay  pipeline=1  pipeline_display=1  ClockPhase=1  use_ena=off  use_sclr=off  allowFloatingPointOverride=on  logOutputs=off  logFile=C:\Workspace\Autotracking\MOSSE_model\tb_MOSSE_HDL_final\MOSSE%5FHDL%5Ffinal_DSP%5FBuilder%5FCompute%5FShift_Delay2.fixedpointlog  use_init=off  reset_value=1
  Divider : allblocks_alteradspbuilder2/Divider  BusType=Unsigned Integer  bwl=12  bwr=0  pipeline=1  pipeline_display=1  use_ena=off  use_aclr=on
  Input : allblocks_alteradspbuilder2/Input  iofile=C:\Workspace\Autotracking\MOSSE_model\tb_MOSSE_HDL_final\MOSSE%5FHDL%5Ffinal_DSP%5FBuilder%5FCompute%5FShift_Input.salt  BusType=Unsigned Integer  bwl=12  bwr=0  SpecifyClock=off  PORTTYPE=Input  externalType=Inferred  allowFloatingPointOverride=on  logOutputs=off
  Input2 : allblocks_alteradspbuilder2/Input  iofile=C:\Workspace\Autotracking\MOSSE_model\tb_MOSSE_HDL_final\MOSSE%5FHDL%5Ffinal_DSP%5FBuilder%5FCompute%5FShift_Input2.salt  BusType=Single Bit  bwl=12  bwr=0  SpecifyClock=off  PORTTYPE=Input  externalType=Inferred  allowFloatingPointOverride=on  logOutputs=off
  Output : allblocks_alteradspbuilder2/Output  iofile=C:\Workspace\Autotracking\MOSSE_model\tb_MOSSE_HDL_final\MOSSE%5FHDL%5Ffinal_DSP%5FBuilder%5FCompute%5FShift_Output.capture  BusType=Signed Integer  bwl=8  bwr=0  externalType=Simulink Fixed Point Type  PORTTYPE=Output  allowFloatingPointOverride=on  logOutputs=off
  Output1 : allblocks_alteradspbuilder2/Output  iofile=C:\Workspace\Autotracking\MOSSE_model\tb_MOSSE_HDL_final\MOSSE%5FHDL%5Ffinal_DSP%5FBuilder%5FCompute%5FShift_Output1.capture  BusType=Signed Integer  bwl=8  bwr=0  externalType=Simulink Fixed Point Type  PORTTYPE=Output  allowFloatingPointOverride=on  logOutputs=off
  Pipelined Adder : allblocks_alteradspbuilder2/Pipelined Adder  BusType=Signed Integer  bwl=12  bwr=0  pipeline=0  pipeline_display=0  AddSubDirection=SUB  use_cin=off  use_ovl=off  use_addsub=off  use_ena=off  use_aclr=off  or_aclr_inputs=on
  Pipelined Adder1 : allblocks_alteradspbuilder2/Pipelined Adder  BusType=Signed Integer  bwl=12  bwr=0  pipeline=0  pipeline_display=0  AddSubDirection=SUB  use_cin=off  use_ovl=off  use_addsub=off  use_ena=off  use_aclr=off  or_aclr_inputs=on
  dx : Outport
  dy : Outport  Port=2
  wires:
  Input/1 -> Divider/1
  Constant/1 -> Divider/2
  In_num/1 -> Input/1
  Output1/1 -> dx/1
  Output/1 -> dy/1
  Divider/1 -> Pipelined Adder/1
  Constant2/1 -> Pipelined Adder1/2
  Pipelined Adder/1 -> Delay/1
  Delay/1 -> Output/1
  Pipelined Adder1/1 -> Delay1/1
  Delay1/1 -> Output1/1
  Divider/2 -> Pipelined Adder1/1
  iaclr/1 -> Input2/1
  Input2/1 -> Delay2/1, Divider/3
  Constant1/1 -> Pipelined Adder/2
  Delay2/1 -> Delay/2, Delay1/2

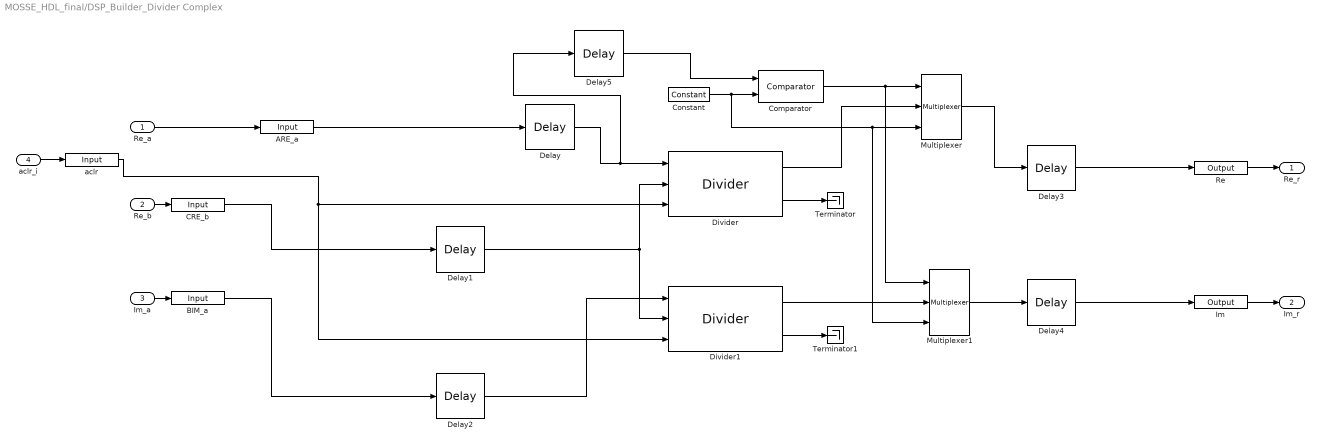
== system MOSSE_HDL_final/DSP_Builder_Divider Complex ==
  Re_a : Inport
  Re_b : Inport  Port=2
  Im_a : Inport  Port=3
  aclr_i : Inport  Port=4
  ARE_a : allblocks_alteradspbuilder2/Input  iofile=E:\Work\ComputerVision\ObjectTrack\MOSSE\autotrackigproject\Model\MOSSE_algorithm\MOSSE_simulink\tb_MOSSE_HDL_final\MOSSE%5FHDL%5Ffinal_DSP%5FBuilder%5FDivider+Complex_ARE%5Fa.salt  BusType=Signed Integer  bwl=32  bwr=0  SpecifyClock=off  PORTTYPE=Input  externalType=Inferred  allowFloatingPointOverride=on  logOutputs=off
  BIM_a : allblocks_alteradspbuilder2/Input  iofile=E:\Work\ComputerVision\ObjectTrack\MOSSE\autotrackigproject\Model\MOSSE_algorithm\MOSSE_simulink\tb_MOSSE_HDL_final\MOSSE%5FHDL%5Ffinal_DSP%5FBuilder%5FDivider+Complex_BIM%5Fa.salt  BusType=Signed Integer  bwl=32  bwr=0  SpecifyClock=off  PORTTYPE=Input  externalType=Inferred  allowFloatingPointOverride=on  logOutputs=off
  CRE_b : allblocks_alteradspbuilder2/Input  iofile=E:\Work\ComputerVision\ObjectTrack\MOSSE\autotrackigproject\Model\MOSSE_algorithm\MOSSE_simulink\tb_MOSSE_HDL_final\MOSSE%5FHDL%5Ffinal_DSP%5FBuilder%5FDivider+Complex_CRE%5Fb.salt  BusType=Signed Integer  bwl=32  bwr=0  SpecifyClock=off  PORTTYPE=Input  externalType=Inferred  allowFloatingPointOverride=on  logOutputs=off
  Comparator : allblocks_alteradspbuilder2/Comparator  direction=a == b  pipeline_display=0  allowFloatingPointOverride=on  logOutputs=off  logFile=E:\Work\ComputerVision\ObjectTrack\MOSSE\autotrackigproject\Model\MOSSE_algorithm\MOSSE_simulink\tb_MOSSE_HDL_final\MOSSE%5FHDL%5Ffinal_DSP%5FBuilder%5FDivider+Complex_Comparator.fixedpointlog
  Constant : allblocks_alteradspbuilder2/Constant  mask_cst=0  BusType=Signed Integer  bwl=32  bwr=0  roundMode=Truncate  satMode=Wrap  SpecifyClock=off  allowFloatingPointOverride=on  logOutputs=off  logFile=E:\Work\ComputerVision\ObjectTrack\MOSSE\autotrackigproject\Model\MOSSE_algorithm\MOSSE_simulink\tb_MOSSE_HDL_final\MOSSE%5FHDL%5Ffinal_DSP%5FBuilder%5FDivider+Complex_Constant.fixedpointlog
  Delay : allblocks_alteradspbuilder2/Delay  pipeline=1  pipeline_display=1  ClockPhase=1  use_ena=off  use_sclr=off  allowFloatingPointOverride=on  logOutputs=off  logFile=E:\Work\ComputerVision\ObjectTrack\MOSSE\autotrackigproject\Model\MOSSE_algorithm\MOSSE_simulink\tb_MOSSE_HDL_final\MOSSE%5FHDL%5Ffinal_DSP%5FBuilder%5FDivider+Complex_Delay.fixedpointlog  use_init=off  reset_value=1
  Delay1 : allblocks_alteradspbuilder2/Delay  pipeline=1  pipeline_display=1  ClockPhase=1  use_ena=off  use_sclr=off  allowFloatingPointOverride=on  logOutputs=off  logFile=E:\Work\ComputerVision\ObjectTrack\MOSSE\autotrackigproject\Model\MOSSE_algorithm\MOSSE_simulink\tb_MOSSE_HDL_final\MOSSE%5FHDL%5Ffinal_DSP%5FBuilder%5FDivider+Complex_Delay1.fixedpointlog  use_init=off  reset_value=1
  Delay2 : allblocks_alteradspbuilder2/Delay  pipeline=1  pipeline_display=1  ClockPhase=1  use_ena=off  use_sclr=off  allowFloatingPointOverride=on  logOutputs=off  logFile=E:\Work\ComputerVision\ObjectTrack\MOSSE\autotrackigproject\Model\MOSSE_algorithm\MOSSE_simulink\tb_MOSSE_HDL_final\MOSSE%5FHDL%5Ffinal_DSP%5FBuilder%5FDivider+Complex_Delay2.fixedpointlog  use_init=off  reset_value=1
  Delay3 : allblocks_alteradspbuilder2/Delay  pipeline=1  pipeline_display=1  ClockPhase=1  use_ena=off  use_sclr=off  allowFloatingPointOverride=on  logOutputs=off  logFile=E:\Work\ComputerVision\ObjectTrack\MOSSE\autotrackigproject\Model\MOSSE_algorithm\MOSSE_simulink\tb_MOSSE_HDL_final\MOSSE%5FHDL%5Ffinal_DSP%5FBuilder%5FDivider+Complex_Delay3.fixedpointlog  use_init=off  reset_value=1
  Delay4 : allblocks_alteradspbuilder2/Delay  pipeline=1  pipeline_display=1  ClockPhase=1  use_ena=off  use_sclr=off  allowFloatingPointOverride=on  logOutputs=off  logFile=E:\Work\ComputerVision\ObjectTrack\MOSSE\autotrackigproject\Model\MOSSE_algorithm\MOSSE_simulink\tb_MOSSE_HDL_final\MOSSE%5FHDL%5Ffinal_DSP%5FBuilder%5FDivider+Complex_Delay4.fixedpointlog  use_init=off  reset_value=1
  Delay5 : allblocks_alteradspbuilder2/Delay  pipeline=4  pipeline_display=4  ClockPhase=1  use_ena=off  use_sclr=off  allowFloatingPointOverride=on  logOutputs=off  logFile=E:\Work\ComputerVision\ObjectTrack\MOSSE\autotrackigproject\Model\MOSSE_algorithm\MOSSE_simulink\tb_MOSSE_HDL_final\MOSSE%5FHDL%5Ffinal_DSP%5FBuilder%5FDivider+Complex_Delay5.fixedpointlog  use_init=off  reset_value=1
  Divider : allblocks_alteradspbuilder2/Divider  BusType=Signed Integer  bwl=32  bwr=0  pipeline=4  pipeline_display=4  use_ena=off  use_aclr=on
  Divider1 : allblocks_alteradspbuilder2/Divider  BusType=Signed Integer  bwl=32  bwr=0  pipeline=4  pipeline_display=4  use_ena=off  use_aclr=on
  Im : allblocks_alteradspbuilder2/Output  iofile=E:\Work\ComputerVision\ObjectTrack\MOSSE\autotrackigproject\Model\MOSSE_algorithm\MOSSE_simulink\tb_MOSSE_HDL_final\MOSSE%5FHDL%5Ffinal_DSP%5FBuilder%5FDivider+Complex_Im.capture  BusType=Signed Integer  bwl=32  bwr=0  externalType=Simulink Fixed Point Type  PORTTYPE=Output  allowFloatingPointOverride=on  logOutputs=off
  Multiplexer : allblocks_alteradspbuilder2/Multiplexer  numInputs=2  pipeline=0  oneHot=off  pipeline_display=0  use_ena=off  use_aclr=off  allowFloatingPointOverride=on  logOutputs=off  logFile=E:\Work\ComputerVision\ObjectTrack\MOSSE\autotrackigproject\Model\MOSSE_algorithm\MOSSE_simulink\tb_MOSSE_HDL_final\MOSSE%5FHDL%5Ffinal_DSP%5FBuilder%5FDivider+Complex_Multiplexer.fixedpointlog
  Multiplexer1 : allblocks_alteradspbuilder2/Multiplexer  numInputs=2  pipeline=0  oneHot=off  pipeline_display=0  use_ena=off  use_aclr=off  allowFloatingPointOverride=on  logOutputs=off  logFile=E:\Work\ComputerVision\ObjectTrack\MOSSE\autotrackigproject\Model\MOSSE_algorithm\MOSSE_simulink\tb_MOSSE_HDL_final\MOSSE%5FHDL%5Ffinal_DSP%5FBuilder%5FDivider+Complex_Multiplexer1.fixedpointlog
  Re : allblocks_alteradspbuilder2/Output  iofile=E:\Work\ComputerVision\ObjectTrack\MOSSE\autotrackigproject\Model\MOSSE_algorithm\MOSSE_simulink\tb_MOSSE_HDL_final\MOSSE%5FHDL%5Ffinal_DSP%5FBuilder%5FDivider+Complex_Re.capture  BusType=Signed Integer  bwl=32  bwr=0  externalType=Simulink Fixed Point Type  PORTTYPE=Output  allowFloatingPointOverride=on  logOutputs=off
  Terminator : Terminator
  Terminator1 : Terminator
  aclr : allblocks_alteradspbuilder2/Input  iofile=E:\Work\ComputerVision\ObjectTrack\MOSSE\autotrackigproject\Model\MOSSE_algorithm\MOSSE_simulink\tb_MOSSE_HDL_final\MOSSE%5FHDL%5Ffinal_DSP%5FBuilder%5FDivider+Complex_aclr.salt  BusType=Single Bit  bwl=32  bwr=0  SpecifyClock=off  PORTTYPE=Input  externalType=Inferred  allowFloatingPointOverride=on  logOutputs=off
  Re_r : Outport
  Im_r : Outport  Port=2
  wires:
  Re/1 -> Re_r/1
  Divider1/2 -> Terminator1/1
  Divider/2 -> Terminator/1
  Re_a/1 -> ARE_a/1
  Re_b/1 -> CRE_b/1
  Im_a/1 -> BIM_a/1
  aclr_i/1 -> aclr/1
  Im/1 -> Im_r/1
  aclr/1 -> Divider/3, Divider1/3
  ARE_a/1 -> Delay/1
  Delay1/1 -> Divider1/2, Divider/2
  CRE_b/1 -> Delay1/1
  Delay2/1 -> Divider1/1
  BIM_a/1 -> Delay2/1
  Delay3/1 -> Re/1
  Delay4/1 -> Im/1
  Divider/1 -> Multiplexer/2
  Multiplexer/1 -> Delay3/1
  Comparator/1 -> Multiplexer1/1, Multiplexer/1
  Constant/1 -> Comparator/2, Multiplexer1/3, Multiplexer/3
  Delay/1 -> Delay5/1, Divider/1
  Delay5/1 -> Comparator/1
  Multiplexer1/1 -> Delay4/1
  Divider1/1 -> Multiplexer1/2
